simulink model "testerdo23"  (R2022b)
settings: Solver=VariableStepAuto  StartTime=0.0  StopTime=10  RelTol=1e-3
values from neighbouring files (symbols this model uses):
  Bv = -[-0.149 0.181]/1000    [dane.m]    (also in tester23.m = [-0.149 0.181]; wykresownik33.m = [-0.149 0.181]; wykresownik35.m = [-0.149 0.181]; wykresownik36.m = [-0.149 0.181])
settings Model: Creator=48519  LastModifiedBy=48519
settings ModelReferenceCC: EnableRefExpFcnMdlSchedulingChecks=on

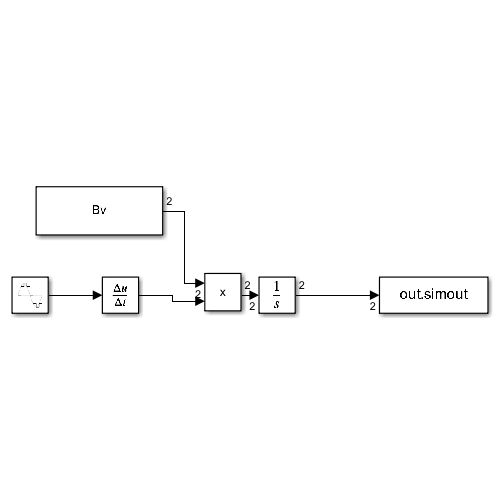
[thumbnail: Simulink's stored preview of the top-level diagram]
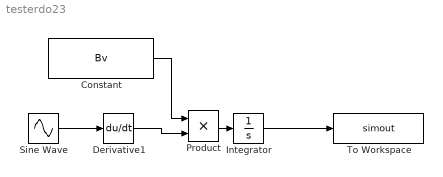
== system testerdo23 ==
  Constant : Constant  Value=Bv
  Derivative1 : Derivative
  Integrator : Integrator  InitialCondition=1
  Product : Product
  Sine Wave : Sin  Amplitude=10  SampleTime=0.01
  To Workspace : ToWorkspace  VariableName=simout  SaveFormat=Timeseries  SampleTime=-1
  wires:
  Sine Wave/1 -> Derivative1/1
  Constant/1 -> Product/1
  Derivative1/1 -> Product/2
  Integrator/1 -> To Workspace/1
  Product/1 -> Integrator/1
